simulink model "SWC_IMU_type"  (R2021b)
settings: Solver=FixedStepDiscrete  StartTime=0.0  StopTime=10.0  RelTol=1e-3
settings Model: DataDictionary=APPTypes.sldd  Creator=FVT23033  LastModifiedBy=FVT23033
settings DataIOCC: SaveFormat=StructureWithTime
settings OptimizationCC: DefaultParameterBehavior=Inlined  EnhancedBackFolding=on  PassReuseOutputArgsAs=Individual arguments  ZeroExternalMemoryAtStartup=off  ZeroInternalMemoryAtStartup=off  OptimizeBlockOrder=speed  DifferentSizesBufferReuse=on  OptimizationCustomize=off  EfficientTunableParamExpr=on
settings DebuggingCC: ParameterTunabilityLossMsg=error
settings HardwareCC: ProdBitPerPointer=32  ProdBitPerSizeT=32  ProdBitPerPtrDiffT=32  ProdLargestAtomicInteger=Long  ProdLargestAtomicFloat=Double  ProdWordSize=32  ProdLongLongMode=on  ProdHWDeviceType=ARM Compatible->ARM Cortex-M
settings SFSimCC: MATLABDynamicMemAlloc=off
settings RTWCC: Description=AUTOSAR  SystemTargetFile=autosar.tlc  GenCodeOnly=on  TemplateMakefile=ert_default_tmf  PortableWordSizes=on
settings CodeAppCC: ForceParamTrailComments=on  IgnoreCustomStorageClasses=off  OperatorAnnotations=on  SimulinkDataObjDesc=on  SFDataObjDesc=on  InsertBlockDesc=on
settings STFCustomTargetCC: TargetLangStandard=C99 (ISO)  MultiwordLength=256  ParMdlRefBuildCompliant=on  CompOptLevelCompliant=on  IncludeMdlTerminateFcn=off  CombineOutputUpdateFcns=on  SuppressErrorStatus=on  ERTCustomFileBanners=on  SupportNonFinite=off  SupportComplex=off  SupportContinuousTime=off  SupportNonInlinedSFcns=off  RemoveResetFunc=on  MATLABClassNameForMDSCustomization=Simulink.SoftwareTarget.ERTCustomization  AutosarCompliant=on  GRTInterface=off  UseToolchainInfoCompliant=on  LookupTableObjectStructAxisOrder=2,1,3,4,...  LUTObjectStructOrderEvenSpacing=Size,Table,Breakpoints  SystemTargetFile=autosar.tlc
settings ERTTargetCC: TargetLangStandard=C99 (ISO)  ConcurrentExecutionCompliant=off  IncludeMdlTerminateFcn=off  SuppressErrorStatus=on  SupportNonFinite=off  SupportComplex=off  ModelStepFunctionPrototypeControlCompliant=off  CPPClassGenCompliant=off  AutosarCompliant=on  LookupTableObjectStructAxisOrder=2,1,3,4,...  LUTObjectStructOrderEvenSpacing=Size,Table,Breakpoints  GenerateASAP2=on  InlinedParameterPlacement=NonHierarchical  ERTCustomFileTemplate=example_file_process.tlc  ConvertIfToSwitch=off  SuppressUnreachableDefaultCases=off  BooleanTrueId=true_MatlabRTW  BooleanFalseId=false_MatlabRTW

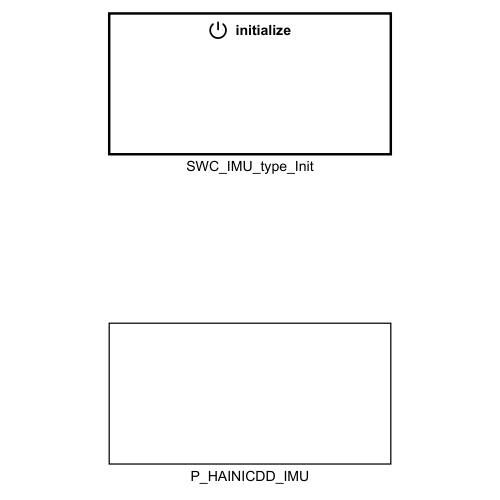
[thumbnail: Simulink's stored preview of the top-level diagram]
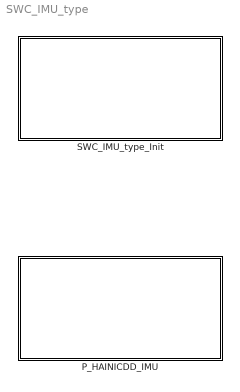
== system SWC_IMU_type ==
  P_HAINICDD_IMU : Subsystem
  SWC_IMU_type_Init : Subsystem

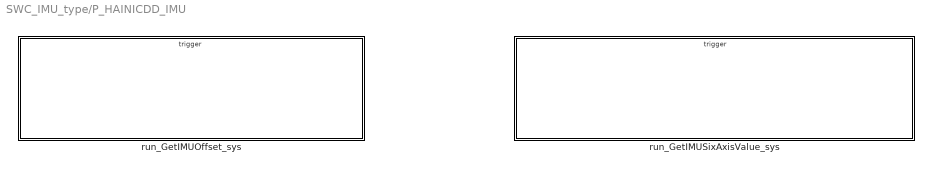
== system SWC_IMU_type/P_HAINICDD_IMU ==
  run_GetIMUOffset_sys : Subsystem
  run_GetIMUSixAxisValue_sys : Subsystem

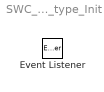
== system SWC_IMU_type/SWC_IMU_type_Init ==
  Event Listener : EventListener  EventName=reset

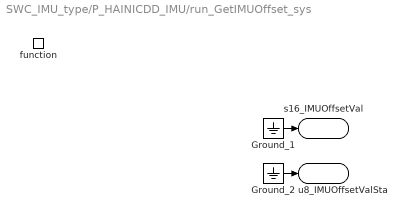
== system SWC_IMU_type/P_HAINICDD_IMU/run_GetIMUOffset_sys ==
  function : TriggerPort  TriggerType=function-call  IsSimulinkFunction=on  FunctionName=run_HALINCDDIMU  VariantControl=(inherit)
  Ground_1 : Ground
  Ground_2 : Ground
  s16_IMUOffsetVal : ArgOut  OutDataTypeStr=int16  PortDimensions=6  ArgumentName=s16_IMUOffsetVal
  u8_IMUOffsetValSta : ArgOut  Port=2  OutDataTypeStr=uint8  ArgumentName=u8_IMUOffsetValSta
  wires:
  Ground_1/1 -> s16_IMUOffsetVal/1
  Ground_2/1 -> u8_IMUOffsetValSta/1

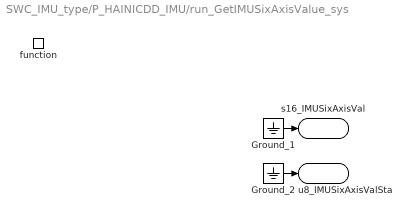
== system SWC_IMU_type/P_HAINICDD_IMU/run_GetIMUSixAxisValue_sys ==
  function : TriggerPort  TriggerType=function-call  IsSimulinkFunction=on  FunctionName=run_GetIMUSixAxisValue  VariantControl=(inherit)
  Ground_1 : Ground
  Ground_2 : Ground
  s16_IMUSixAxisVal : ArgOut  OutDataTypeStr=int16  PortDimensions=6  ArgumentName=s16_IMUSixAxisVal
  u8_IMUSixAxisValSta : ArgOut  Port=2  OutDataTypeStr=uint8  ArgumentName=u8_IMUSixAxisValSta
  wires:
  Ground_1/1 -> s16_IMUSixAxisVal/1
  Ground_2/1 -> u8_IMUSixAxisValSta/1
